simulink model "lab4_1z"  (R2023b)
settings: Solver=FixedStepAuto  StartTime=0.0  StopTime=10.0  FixedStep=0.001  RelTol=1e-3
undefined symbols (not defined in the file): a_0, a_1, a_2, k_0, k_1
settings Model: Creator=nsukh  LastModifiedBy=nsukh

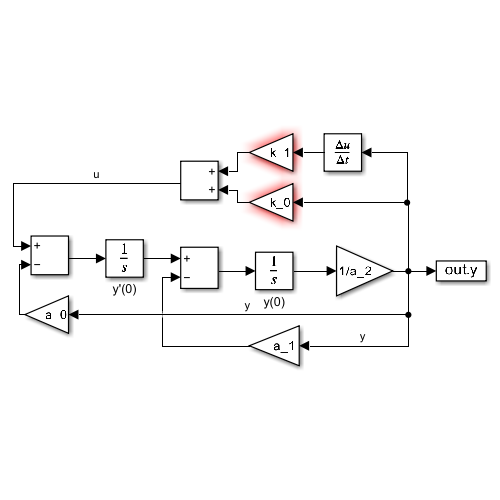
[thumbnail: Simulink's stored preview of the top-level diagram]
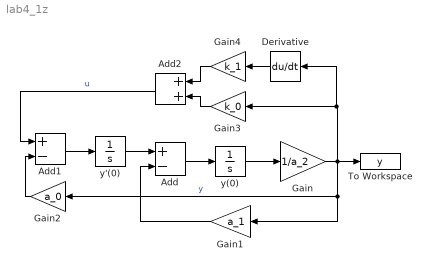
== system lab4_1z ==
  Add : Sum  Inputs=+-
  Add1 : Sum  Inputs=+-
  Add2 : Sum
  Derivative : Derivative
  Gain : Gain  Gain=1/a_2
  Gain1 : Gain  Gain=a_1
  Gain2 : Gain  Gain=a_0
  Gain3 : Gain  Gain=k_0
  Gain4 : Gain  Gain=k_1
  To Workspace : ToWorkspace  VariableName=y  SaveFormat=Timeseries  SampleTime=-1
  y'(0) : Integrator  InitialCondition=4
  y(0) : Integrator
  wires:
  y(0)/1 -> Gain/1
  Gain/1 -> Derivative/1, Gain3/1, To Workspace/1, Gain1/1, Gain2/1  "y"
  Add/1 -> y(0)/1
  Gain1/1 -> Add/2
  y'(0)/1 -> Add/1
  Add1/1 -> y'(0)/1
  Add2/1 -> Add1/1  "u"
  Gain2/1 -> Add1/2
  Gain3/1 -> Add2/2
  Derivative/1 -> Gain4/1
  Gain4/1 -> Add2/1
